simulink model "Motor_Speed_closedloop"  (Simulink 8.3)
settings: Solver=ode45  StartTime=0.0  StopTime=10.0  RelTol=1e-3
undefined symbols (not defined in the file or in its folder): b, J, K, L, R
settings Model: Creator=maen  LastModifiedBy=JATIN
settings OptimizationCC: ExpressionDepthLimit=2147483647
settings DebuggingCC: SolverPrmCheckMsg=none  FcnCallInpInsideContextMsg=UseLocalSettings
settings ConfigurationSet: Description=SimMechanics 2G

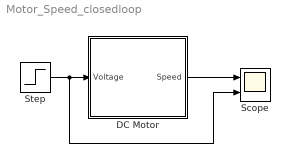
== system Motor_Speed_closedloop ==
  DC Motor : Subsystem
  Scope : Scope  NumInputPorts=2
      settings: TimeRange=0.2  YMin=0~-5  YMax=10~5
  Step : Step  Time=0  SampleTime=0
  wires:
  Step/1 -> Scope/2, DC Motor/1(Voltage)
  DC Motor/1(" Speed") -> Scope/1

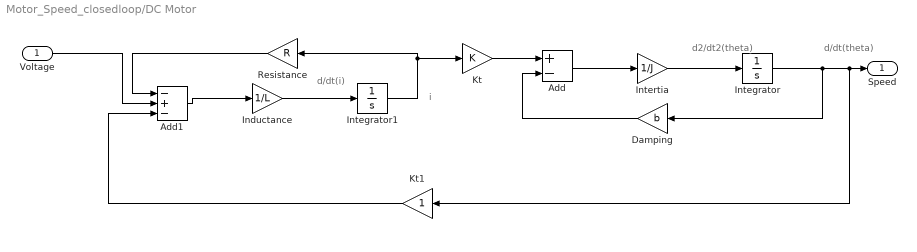
== system Motor_Speed_closedloop/DC Motor ==
  note: i
  note: d/dt(theta)
  note: d2/dt2(theta)
  note: d/dt(i)
  Voltage : Inport
  Add : Sum  Inputs=+-
  Add1 : Sum  Inputs=-+-
  Damping : Gain  Gain=b
  Inductance : Gain  Gain=1/L
  Integrator : Integrator
  Integrator1 : Integrator
  Intertia : Gain  Gain=1/J
  Kt : Gain  Gain=K
  Kt1 : Gain
  Resistance : Gain  Gain=R
  " Speed" : Outport
  wires:
  Integrator1/1 -> Kt/1, Resistance/1
  Inductance/1 -> Integrator1/1
  Intertia/1 -> Integrator/1
  Integrator/1 -> Damping/1, Kt1/1, " Speed"/1
  Add1/1 -> Inductance/1
  Add/1 -> Intertia/1
  Damping/1 -> Add/2
  Kt/1 -> Add/1
  Resistance/1 -> Add1/1
  Voltage/1 -> Add1/2
  Kt1/1 -> Add1/3
